simulink model "RevisedOrbitFollowing"  (R2015b)
settings: Solver=VariableStepAuto  StartTime=0.0  StopTime=1000  FixedStep=0.001  RelTol=1e-9
values from neighbouring files (symbols this model uses):
  A = 3    [RevisedMethod.m]
  alpha = 1.65    [BeardMethod.m]    (also in OrbitCenter.m = abs((ang1-ang2)/2); RevisedMethod.m)
  course_int = course_int+2*pi    (= 6.28318530718)    [BeardMethod.m]    (also in RevisedMethod.m = -0.785398163397)
  cx = C(1)    [BeardMethod.m]    (also in RevisedMethod.m = 50)
  cy = C(2)    [BeardMethod.m]    (also in RevisedMethod.m = 50)
  d_int = norm([x.data(end),y.data(end)]-[cx,cy])    [BeardMethod.m]    (also in RevisedMethod.m = 15)
  epsi = 0.1    [BeardMethod.m]    (also in RevisedMethod.m = 0.5)
  Gamma = 80    [RevisedMethod.m]
  gamma_end = (pi+(pi/2-2*alpha))    [OrbitCenter.m]    (also in RevisedMethod.m = 47.1238898038)
  gamma_int = atan2((y.data(end)-cy),(x.data(end)-cx))    [BeardMethod.m]    (also in RevisedMethod.m = 0.785398163397)
  j = Rotation(i)    [BeardMethod.m]    (also in RevisedMethod.m = -1)
  k = 0.02    [BeardMethod.m]    (also in RevisedMethod.m = 0.1)
  kk = pi/2    (= 1.57079632679)    [BeardMethod.m]    (also in RevisedMethod.m)
  Method = 3    [RevisedMethod.m]
  phiA = pi    (= 3.14159265359)    [RevisedMethod.m]
  phiw = 230/180*pi    (= 4.01425727959)    [BeardMethod.m]    (also in RevisedMethod.m)
  R = 10    [BeardMethod.m]    (also in RevisedMethod.m)
  Va = 13    [BeardMethod.m]    (also in RevisedMethod.m)
  Vg0 = sqrt((Va*sin(phi)+W*sin(phiw))^2+(Va*cos(phi)+W*cos(phiw))^2)    [InitialVg.m]    (also in RevisedMethod.m = InitialVg(A,0,W,phiw,Va,course_int))
  W = 6    [RevisedMethod.m]
libraries: simulink x1
settings Model: Creator=Bingyu Zhou  LastModifiedBy=Bingyu Zhou

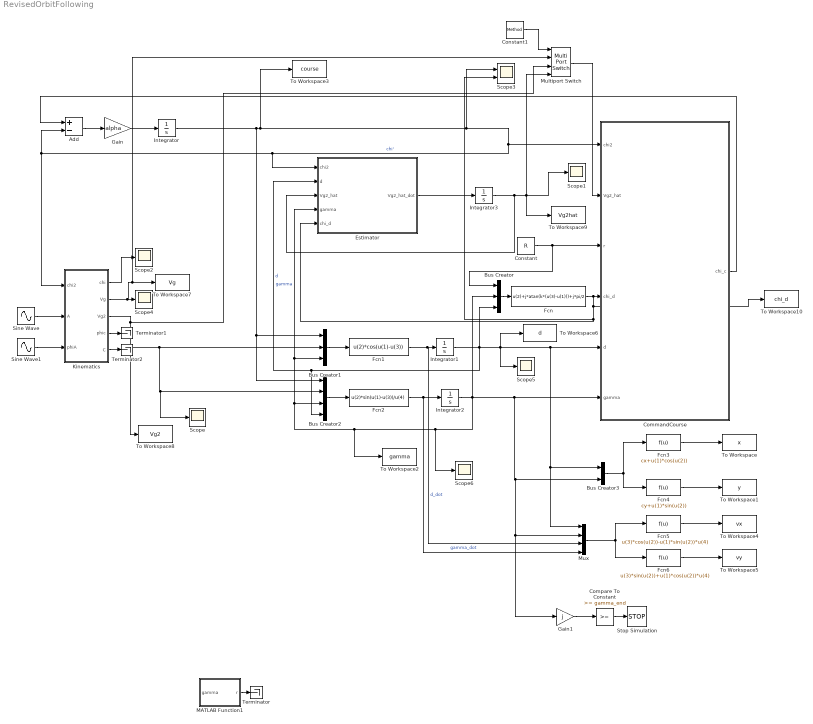
== system RevisedOrbitFollowing ==
  Add : Sum  Inputs=+-
  Bus Creator : BusCreator  Inputs=3
  Bus Creator1 : BusCreator  Inputs=3
  Bus Creator2 : BusCreator  Inputs=4
  Bus Creator3 : BusCreator  Inputs=2
  CommandCourse : Subsystem
  Compare To Constant : simulink/Logic and Bit Operations/Compare To Constant  relop=>=  const=gamma_end  OutDataTypeStr=boolean
  Constant : Constant  Value=R
  Constant1 : Constant  Value=Method
  "Estimator " : MATLAB Function  TreatAsAtomicUnit=on
  Fcn : Fcn  Expr=u(2)+j*atan(k*(u(3)-u(1)))+j*pi/2
  Fcn1 : Fcn  Expr=u(2)*cos(u(1)-u(3))
  Fcn2 : Fcn  Expr=u(2)*sin(u(1)-u(3))/u(4)
  Fcn3 : Fcn  Expr=cx+u(1)*cos(u(2))
  Fcn4 : Fcn  Expr=cy+u(1)*sin(u(2))
  Fcn5 : Fcn  Expr=u(3)*cos(u(2))-u(1)*sin(u(2))*u(4)
  Fcn6 : Fcn  Expr=u(3)*sin(u(2))+u(1)*cos(u(2))*u(4)
  Gain : Gain  Gain=alpha
  Gain1 : Gain  Gain=j
  Integrator : Integrator  InitialCondition=course_int
  Integrator1 : Integrator  InitialCondition=d_int
  Integrator2 : Integrator  InitialCondition=gamma_int  WrappedStateUpperValue=0  WrappedStateLowerValue=-2*pi
  Integrator3 : Integrator  InitialCondition=Vg0
  Kinematics : Subsystem
  MATLAB Function1 : MATLAB Function  TreatAsAtomicUnit=on
  Multiport Switch : MultiPortSwitch
  Mux : Mux
  Scope{,1..2,4..6} (6 alike) : Scope
  Scope3 : Scope  NumInputPorts=2
  Sine Wave : Sin  Amplitude=A  Frequency=0.1  Phase=pi/2  SampleTime=0
  Sine Wave1 : Sin  Amplitude=phiA  Frequency=0.1  SampleTime=0
  Stop Simulation : Stop
  Terminator : Terminator
  Terminator1 : Terminator
  Terminator2 : Terminator
  To Workspace : ToWorkspace  VariableName=x  SaveFormat=Timeseries  SampleTime=-1
  To Workspace1 : ToWorkspace  VariableName=y  SaveFormat=Timeseries  SampleTime=-1
  To Workspace10 : ToWorkspace  VariableName=chi_d  SaveFormat=Timeseries  SampleTime=-1
  To Workspace2 : ToWorkspace  VariableName=gamma  SaveFormat=Timeseries  SampleTime=-1
  To Workspace3 : ToWorkspace  VariableName=course  SaveFormat=Timeseries  SampleTime=-1
  To Workspace4 : ToWorkspace  VariableName=vx  SaveFormat=Timeseries  SampleTime=-1
  To Workspace5 : ToWorkspace  VariableName=vy  SaveFormat=Timeseries  SampleTime=-1
  To Workspace6 : ToWorkspace  VariableName=d  SaveFormat=Timeseries  SampleTime=-1
  To Workspace7 : ToWorkspace  VariableName=Vg  SaveFormat=Timeseries  SampleTime=-1
  To Workspace8 : ToWorkspace  VariableName=Vg2  SaveFormat=Timeseries  SampleTime=-1
  To Workspace9 : ToWorkspace  VariableName=Vg2hat  SaveFormat=Timeseries  SampleTime=-1
  wires:
  Add/1 -> Gain/1
  Gain/1 -> Integrator/1
  Integrator/1 -> To Workspace3/1, Scope3/1, CommandCourse/1(chi2), "Estimator "/1(chi2), Kinematics/1(chi2), Add/2, Bus Creator2/1, Bus Creator1/1  "chi'"
  Bus Creator/1 -> Fcn/1
  Bus Creator1/1 -> Fcn1/1
  Fcn1/1 -> Mux/3, Integrator1/1  "d_dot"
  Fcn2/1 -> Mux/4, Integrator2/1  "gamma_dot"
  Integrator2/1 -> Bus Creator/2, Mux/2, Gain1/1, Bus Creator3/2, CommandCourse/6(gamma), Scope6/1, To Workspace2/1, "Estimator "/4(gamma), Bus Creator1/3, Bus Creator2/3  "gamma"
  Bus Creator2/1 -> Fcn2/1
  Integrator1/1 -> Bus Creator/3, "Estimator "/2(d), Bus Creator2/4, To Workspace6/1, Scope5/1, Mux/1, Bus Creator3/1, CommandCourse/5(d)  "d"
  Fcn/1 -> "Estimator "/5(chi_d), Scope3/2, To Workspace10/1, CommandCourse/4(chi_d)
  Bus Creator3/1 -> Fcn3/1, Fcn4/1
  Fcn3/1 -> To Workspace/1
  Fcn4/1 -> To Workspace1/1
  CommandCourse/1(chi_c) -> Add/1
  Constant/1 -> Bus Creator/1, CommandCourse/3("r ")
  MATLAB Function1/1(r) -> Terminator/1
  Kinematics/3(Vg2) -> Multiport Switch/3, To Workspace8/1, Scope/1, Bus Creator2/2, Bus Creator1/2
  "Estimator "/1(Vg2_hat_dot) -> Integrator3/1
  Integrator3/1 -> "Estimator "/3(Vg2_hat), Multiport Switch/4, To Workspace9/1, Scope1/1
  Kinematics/2(Vg) -> Multiport Switch/2, To Workspace7/1, Scope4/1
  Compare To Constant/1 -> Stop Simulation/1
  Gain1/1 -> Compare To Constant/1
  Mux/1 -> Fcn6/1, Fcn5/1
  Fcn5/1 -> To Workspace4/1
  Fcn6/1 -> To Workspace5/1
  Kinematics/1(chi) -> Scope2/1
  Sine Wave/1 -> Kinematics/2(A)
  Sine Wave1/1 -> Kinematics/3(phiA)
  Kinematics/4(phic) -> Terminator1/1
  Kinematics/5(C) -> Terminator2/1
  Multiport Switch/1 -> CommandCourse/2(Vg2_hat)
  Constant1/1 -> Multiport Switch/1

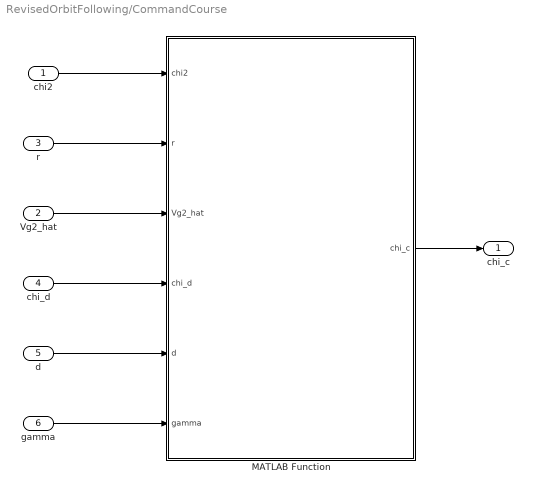
== system RevisedOrbitFollowing/CommandCourse ==
  chi2 : Inport
  Vg2_hat : Inport  Port=2
  "r " : Inport  Port=3
  chi_d : Inport  Port=4
  d : Inport  Port=5
  gamma : Inport  Port=6
  MATLAB Function : MATLAB Function  TreatAsAtomicUnit=on
  chi_c : Outport
  wires:
  chi_d/1 -> MATLAB Function/4(chi_d)
  Vg2_hat/1 -> MATLAB Function/3(Vg2_hat)
  chi2/1 -> MATLAB Function/1(chi2)
  MATLAB Function/1(chi_c) -> chi_c/1
  "r "/1 -> MATLAB Function/2(r)
  d/1 -> MATLAB Function/5(d)
  gamma/1 -> MATLAB Function/6(gamma)

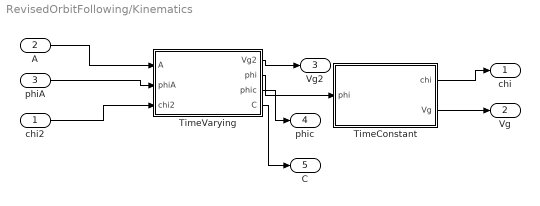
== system RevisedOrbitFollowing/Kinematics ==
  chi2 : Inport
  A : Inport  Port=2
  phiA : Inport  Port=3
  TimeConstant : MATLAB Function  TreatAsAtomicUnit=on
  TimeVarying : MATLAB Function  TreatAsAtomicUnit=on
  chi : Outport
  Vg : Outport  Port=2
  Vg2 : Outport  Port=3
  phic : Outport  Port=4
  C : Outport  Port=5
  wires:
  A/1 -> TimeVarying/1(A)
  TimeVarying/2(phi) -> TimeConstant/1(phi)
  TimeConstant/2(Vg) -> Vg/1
  phiA/1 -> TimeVarying/2(phiA)
  TimeConstant/1(chi) -> chi/1
  chi2/1 -> TimeVarying/3(chi2)
  TimeVarying/1(Vg2) -> Vg2/1
  TimeVarying/3(phic) -> phic/1
  TimeVarying/4(C) -> C/1

== matlab function RevisedOrbitFollowing/Estimator  ==
  data: chi2 input; d input; Vg2_hat_dot output; Vg2_hat input; gamma input; chi_d input; W parameter; phiw parameter; Va parameter; k parameter; kk parameter; epsi parameter; d_int parameter; R parameter; j parameter; Gamma parameter
function Vg2_hat_dot = estimator(chi2,d,Vg2_hat,gamma,chi_d,W,phiw,Va,k,kk,epsi,d_int,R,j,Gamma)
%estimator of Vg'
term = (chi2-chi_d)/epsi;
rho = d_int^2/pi^2;

if abs(term)<=1
    sat = term;
else
    sat = sign(term);
end
% partial derivative of Vg' over chi'
beta = k/(1+(k*(d-R))^2);
der = W*sin(phiw-chi2)+(Va^2-W^2*(sin(phiw-chi2))^2)^(-0.5)*W^2*sin(phiw-chi2)*cos(phiw-chi2); 

Vg2_hat_dot = der*(Vg2_hat*sin(chi2-gamma)/d+j*beta*Vg2_hat*cos(chi2-gamma)-kk*sat)-Gamma*rho*(chi2-chi_d)*(j*beta*cos(chi2-gamma)+sin(chi2-gamma)/d);

end

== matlab function RevisedOrbitFollowing/CommandCourse/MATLAB Function ==
  data: chi2 input; r input; chi_c output; Vg2_hat input; chi_d input; d input; gamma input; epsi parameter; alpha parameter; k parameter; kk parameter; j parameter
function chi_c = CommandCourse(chi2,r,Vg2_hat,chi_d,d,gamma,epsi,alpha,k,kk,j)
%generate course angle for orbit following
term = (chi2-chi_d)/epsi;
if abs(term)<=1
    sat = term;
else
    sat = sign(term);
end
beta = k/(1+(k*(d-r))^2);
chi_c = chi2+Vg2_hat/alpha/d*sin(chi2-gamma)+j*beta/alpha*Vg2_hat*cos(chi2-gamma)-kk/alpha*sat;
end

== matlab function RevisedOrbitFollowing/MATLAB Function1 ==
  data: gamma input; r output
function r = radius(gamma)
%#codegen
if abs(gamma)<=4*pi
    r=70;
else
    r=50;
end
end

== matlab function RevisedOrbitFollowing/Kinematics/TimeConstant ==
  data: phi input; chi output; Va parameter; W parameter; phiw parameter; Vg output
function [chi,Vg] = TimeConstant(phi,Va,W,phiw)
%calculation of Vg and chi

chi = atan2(Va*sin(phi)+W*sin(phiw),Va*cos(phi)+W*cos(phiw));
Vg = sqrt((Va*sin(phi)+W*sin(phiw))^2+(Va*cos(phi)+W*cos(phiw))^2);

end

== matlab function RevisedOrbitFollowing/Kinematics/TimeVarying ==
  data: A input; phiA input; W parameter; phiw parameter; chi2 input; Va parameter; Vg2 output; phi output; phic output; C output
function [Vg2,phi,phic,C] = TimeVarying(A,phiA,W,phiw,chi2,Va)
%Calculation of Vg' and phi (heading angle) based on velocity projection on
%x,y axis.

% Combine the constant and time varying part of current
% C cos(phic) = W cos(phiw)+ A cos(phiA)
% C sin(phic) = W sin(phiw)+ A sin(phiA)
phic = atan2(W*sin(phiw)+A*sin(phiA),W*cos(phiw)+A*cos(phiA));
C = sqrt((W*sin(phiw)+A*sin(phiA))^2+(W*cos(phiw)+A*cos(phiA))^2);

%Calculate Vg' and phi based on Va and C
%Vg' cos(X') = Va cos(phi) + C cos(phic)
%Vg' sin(X') = Va sin(phi) + C sin(phic)
Vg2 = C*cos(phic-chi2)+sqrt(Va^2-C^2*sin(phic-chi2)^2);
phi = atan2(-C/Va*sin(phic-chi2),sqrt(1-C^2/Va^2*sin(phic-chi2)^2))+chi2;
end
